simulink model "fuzzy_impedence_control_Final"  (R2018b)
settings: Solver=VariableStepAuto  StartTime=0.0  StopTime=20  RelTol=1e-3
libraries: fuzblock x2
settings Model: Creator=vojislav  LastModifiedBy=Nick

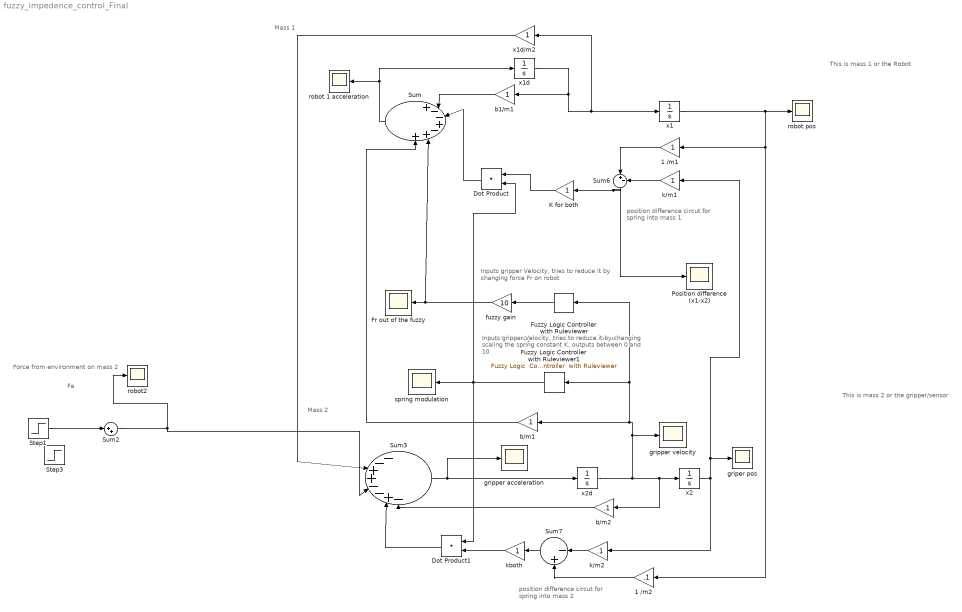
== system fuzzy_impedence_control_Final ==
  note: This is mass 1 or the Robot
  note: position difference circut
      | for spring into mass 1
  note: Inputs gripper Velocity, tries to reduce
      | it by changing force Fr on robot
  note: Fe
  note: Force from environment
      | on mass 2
  note: Mass 1
  note: Mass 2
  note: position difference circut
      | for spring into mass 2
  note: This is mass 2 or the gripper/sensor
  note: Inputs gripper Velocity, tries to reduce
      | it by changing scaling the spring constant
      | K, outputs between 0 and 10
  1 /m1 : Gain
  1 /m2 : Gain  Gain=.1
  Dot Product : DotProduct  InputSameDT=on  OutDataTypeStr=Inherit: Inherit via internal rule
  Dot Product1 : DotProduct  InputSameDT=on  OutDataTypeStr=Inherit: Inherit via internal rule
  "Fr out of the fuzzy " : Scope
  Fuzzy Logic Controller with Ruleviewer : fuzblock/Fuzzy Logic  Controller  with Ruleviewer  fismatrix=fuzzyForceerrorwider  Ts=.25
  Fuzzy Logic Controller with Ruleviewer1 : fuzblock/Fuzzy Logic  Controller  with Ruleviewer  fismatrix=fuzzyKerror  Ts=.25
  "K for both " : Gain
  Position difference (x1-x2) : Scope
  Step1 : Step  Time=0  After=.1  SampleTime=0
  Step3 : Step  Time=4  After=-1  SampleTime=0
  Sum : Sum  Inputs=|+--+-++
  Sum2 : Sum  Inputs=|++
  Sum3 : Sum  Inputs=|--++--+-
  Sum6 : Sum  Inputs=|+-
  Sum7 : Sum  Inputs=|-+
  b/m1 : Gain
  b/m2 : Gain  Gain=.1
  b1/m1 : Gain
  fuzzy gain : Gain  Gain=10
  griper pos : Scope
  gripper acceleration : Scope
  gripper velocity : Scope
  k/m1 : Gain
  k/m2 : Gain  Gain=.1
  "kboth " : Gain
  robot 1 acceleration : Scope
  robot pos : Scope
  robot2 : Scope
  spring modulation : Scope
  x1 : Integrator
  x1d : Integrator
  x1d/m2 : Gain
  x2 : Integrator
  x2d : Integrator  InitialCondition=-1
  wires:
  Sum/1 -> robot 1 acceleration/1, x1d/1
  x1d/1 -> x1/1, x1d/m2/1, b1/m1/1
  Sum3/1 -> x2d/1, gripper acceleration/1
  x2d/1 -> gripper velocity/1, Fuzzy Logic Controller with Ruleviewer/1, Fuzzy Logic Controller with Ruleviewer1/1, b/m1/1, x2/1, b/m2/1
  x1/1 -> 1 /m2/1, 1 /m1/1, robot pos/1
  Step1/1 -> Sum2/1
  Sum2/1 -> Sum3/5, robot2/1
  x2/1 -> k/m1/1, griper pos/1, k/m2/1
  1 /m1/1 -> Sum6/1
  k/m1/1 -> Sum6/2
  k/m2/1 -> Sum7/1
  Sum7/1 -> "kboth "/1
  b/m1/1 -> Sum/7
  1 /m2/1 -> Sum7/2
  b/m2/1 -> Sum3/8
  x1d/m2/1 -> Sum3/3
  Sum6/1 -> Position difference (x1-x2)/1, "K for both "/1
  b1/m1/1 -> Sum/2
  Fuzzy Logic Controller with Ruleviewer/1 -> fuzzy gain/1
  fuzzy gain/1 -> Sum/6, "Fr out of the fuzzy "/1
  "K for both "/1 -> Dot Product/1
  Dot Product/1 -> Sum/3
  "kboth "/1 -> Dot Product1/2
  Dot Product1/1 -> Sum3/7
  Fuzzy Logic Controller with Ruleviewer1/1 -> spring modulation/1, Dot Product/2, Dot Product1/1
